simulink model "scheme6"  (R2024a)
settings: Solver=VariableStepAuto  StartTime=0.0  StopTime=100  RelTol=1e-3
values from neighbouring files (symbols this model uses):
  func = sin_node(A, 0.25)    [main.m]
settings Model: Creator=alexivanov  LastModifiedBy=alexivanov

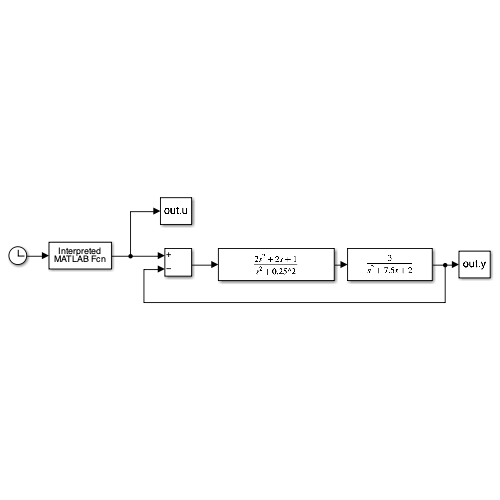
[thumbnail: Simulink's stored preview of the top-level diagram]
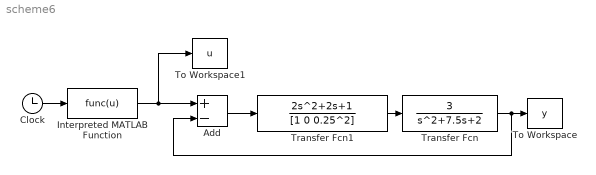
== system scheme6 ==
  Add : Sum  Inputs=+-
  Clock : Clock
  Interpreted MATLAB Function : MATLABFcn  MATLABFcn=func(u)
  To Workspace : ToWorkspace  VariableName=y  SaveFormat=Timeseries  SampleTime=-1
  To Workspace1 : ToWorkspace  VariableName=u  SaveFormat=Timeseries  SampleTime=-1
  Transfer Fcn : TransferFcn  Numerator=[3]  Denominator=[1 7.5 2]
  Transfer Fcn1 : TransferFcn  Numerator=[2 2 1]  Denominator=[1 0 0.25^2]
  wires:
  Clock/1 -> Interpreted MATLAB Function/1
  Interpreted MATLAB Function/1 -> Add/1, To Workspace1/1
  Transfer Fcn/1 -> Add/2, To Workspace/1
  Transfer Fcn1/1 -> Transfer Fcn/1
  Add/1 -> Transfer Fcn1/1
